simulink model "as_workflow"  (R2021b)
settings: Solver=FixedStepDiscrete  StartTime=0.0  StopTime=inf  FixedStep=0.1  RelTol=1e-3  EnableMultiTasking=on
model workspace (MAT data in the model file):
  Numeric = Simulink.NumericType
  Numeric.DataTypeMode = 'Double'
  Numeric.SignednessBool = 1
  Numeric.WordLength = 64
  Numeric.FixedExponent = 0
  Numeric.SlopeAdjustmentFactor = 1
  Numeric.Bias = 0
  Numeric.DataTypeOverride = 'Inherit'
  Numeric.IsAlias = 1
  Numeric.DataScope = 'Auto'
  Param = Simulink.Parameter
  Param.DataType = 'auto'
  Param.Complexity = 'real'
  Param.Dimensions = [0 0]
  Var = 0
settings Model: DataDictionary=data_state.sldd  Creator=altrof  LastModifiedBy=altrof
settings SolverCC: AlgebraicLoopSolver=TrustRegion  AutoInsertRateTranBlk=on
settings DataIOCC: LimitDataPoints=on
settings OptimizationCC: DefaultParameterBehavior=Inlined  EnhancedBackFolding=on  PassReuseOutputArgsAs=Individual arguments  ZeroExternalMemoryAtStartup=off  ZeroInternalMemoryAtStartup=off  OptimizeBlockOrder=speed  DifferentSizesBufferReuse=on  OptimizationCustomize=off  EfficientTunableParamExpr=on
settings DebuggingCC: ParameterTunabilityLossMsg=error  AllowSymbolicDim=off  SFUnexpectedBacktrackingDiag=warning  SFNoUnconditionalDefaultTransitionDiag=warning  SFExecutionAtInitializationDiag=none  ArithmeticOperatorsInVariantConditions=warning
settings SFSimCC: SimUseLocalCustomCode=off  SimDebugExecutionForCustomCode=on  MATLABDynamicMemAlloc=off  CustomCodeUndefinedFunction=UseInterfaceOnly  CustomCodeGlobalsAsFunctionIO=on  DefaultCustomCodeDeterministicFunctions=All  SimTargetLang=C++
settings RTWCC: Description=Embedded Coder  SystemTargetFile=ert.tlc  GenCodeOnly=on  TemplateMakefile=ert_default_tmf  RTWUseLocalCustomCode=off  TargetLang=C++
settings CodeAppCC: ForceParamTrailComments=on  IgnoreCustomStorageClasses=off  OperatorAnnotations=on  SimulinkDataObjDesc=on  SFDataObjDesc=on  InsertBlockDesc=on  UseSimReservedNames=on
settings ERTTargetCC: TargetLangStandard=C++11 (ISO)  GenerateSampleERTMain=on  CodeInterfacePackaging=C++ class  InlinedParameterPlacement=NonHierarchical  RootIOFormat=Structure reference  ERTCustomFileTemplate=example_file_process.tlc
settings ConfigComp: CovMetricSettings=dw  CovSaveCumulativeToWorkspaceVar=on  CovSaveSingleToWorkspaceVar=on  CovExternalEMLEnable=off  CovSFcnEnable=off

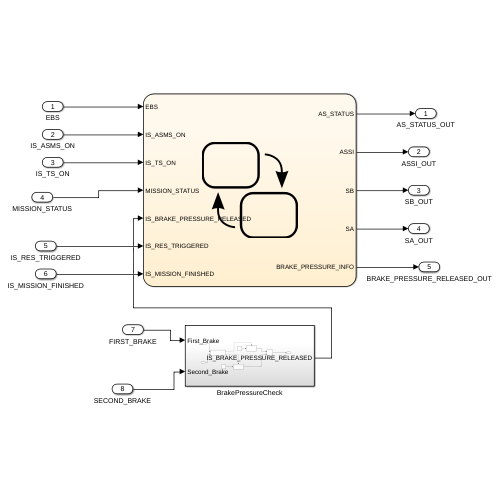
[thumbnail: Simulink's stored preview of the top-level diagram]
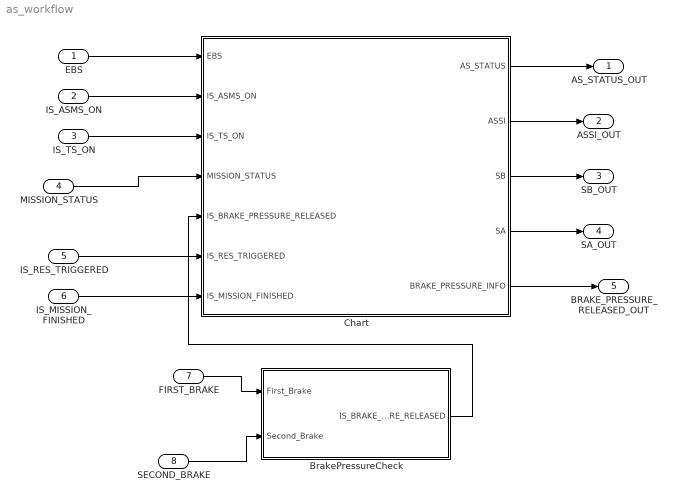
== system as_workflow ==
  EBS : Inport
  IS_ASMS_ON : Inport  Port=2
  IS_TS_ON : Inport  Port=3
  MISSION_STATUS : Inport  Port=4
  IS_RES_TRIGGERED : Inport  Port=5  OutDataTypeStr=boolean
  IS_MISSION_FINISHED : Inport  Port=6  OutDataTypeStr=boolean
  FIRST_BRAKE : Inport  Port=7  OutDataTypeStr=double
  SECOND_BRAKE : Inport  Port=8  OutDataTypeStr=double
  BrakePressureCheck : Subsystem
  Chart : Stateflow chart  TreatAsAtomicUnit=on
  AS_STATUS_OUT : Outport
  ASSI_OUT : Outport  Port=2
  SB_OUT : Outport  Port=3
  SA_OUT : Outport  Port=4
  BRAKE_PRESSURE_RELEASED_OUT : Outport  Port=5
  wires:
  MISSION_STATUS/1 -> Chart/4(MISSION_STATUS)
  EBS/1 -> Chart/1(EBS)
  Chart/1(AS_STATUS) -> AS_STATUS_OUT/1
  Chart/2(ASSI) -> ASSI_OUT/1
  Chart/4(SA) -> SA_OUT/1
  Chart/3(SB) -> SB_OUT/1
  BrakePressureCheck/1(IS_BRAKE_PRESSURE_RELEASED) -> Chart/5(IS_BRAKE_PRESSURE_RELEASED)
  FIRST_BRAKE/1 -> BrakePressureCheck/1(First_Brake)
  SECOND_BRAKE/1 -> BrakePressureCheck/2(Second_Brake)
  Chart/5(BRAKE_PRESSURE_INFO) -> BRAKE_PRESSURE_RELEASED_OUT/1
  IS_RES_TRIGGERED/1 -> Chart/6(IS_RES_TRIGGERED)
  IS_MISSION_FINISHED/1 -> Chart/7(IS_MISSION_FINISHED)
  IS_ASMS_ON/1 -> Chart/2(IS_ASMS_ON)
  IS_TS_ON/1 -> Chart/3(IS_TS_ON)

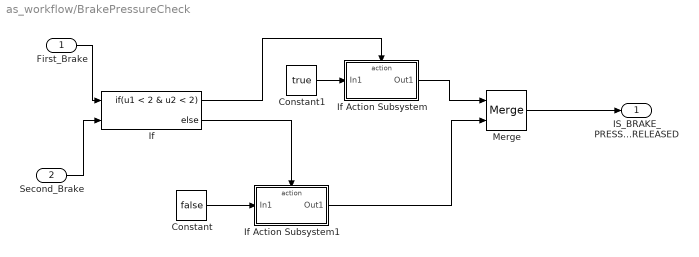
== system as_workflow/BrakePressureCheck ==
  First_Brake : Inport  OutDataTypeStr=double  PortDimensions=1
  Second_Brake : Inport  Port=2  OutDataTypeStr=double  PortDimensions=1
  Constant : Constant  Value=false  OutDataTypeStr=boolean
  Constant1 : Constant  Value=true  OutDataTypeStr=boolean
  If : If  NumInputs=2  IfExpression=u1 < 2 & u2 < 2
  If Action Subsystem : Subsystem  TreatAsAtomicUnit=on
  If Action Subsystem1 : Subsystem  TreatAsAtomicUnit=on
  Merge : Merge
  IS_BRAKE_PRESSURE_RELEASED : Outport
  wires:
  If/1 -> If Action Subsystem/Action
  If/2 -> If Action Subsystem1/Action
  Merge/1 -> IS_BRAKE_PRESSURE_RELEASED/1
  Second_Brake/1 -> If/2
  First_Brake/1 -> If/1
  If Action Subsystem/1(Out1) -> Merge/1
  If Action Subsystem1/1(Out1) -> Merge/2
  Constant/1 -> If Action Subsystem1/1(In1)
  Constant1/1 -> If Action Subsystem/1(In1)

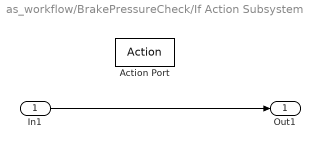
== system as_workflow/BrakePressureCheck/If Action Subsystem ==
  In1 : Inport
  Action Port : ActionPort  ActionPortLabel=if(u1 < 2 & u2 < 2)
  Out1 : Outport
  wires:
  In1/1 -> Out1/1

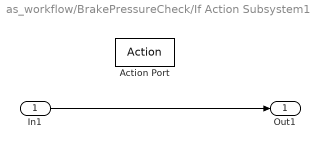
== system as_workflow/BrakePressureCheck/If Action Subsystem1 ==
  In1 : Inport
  Action Port : ActionPort  ActionPortLabel=else
  Out1 : Outport
  wires:
  In1/1 -> Out1/1

== stateflow chart as_workflow/Chart ==
  state AS_READY
    during:
    AS_STATUS = AS_STATE.AS_READY
    SA = SA_STATE.AVAILABLE;
    SB = SB_STATE.ENGAGED;
    ASSI = ASSI_STATE.READY;
  state AS_DRIVING
    during:
    AS_STATUS = AS_STATE.AS_DRIVING
    SA = SA_STATE.AVAILABLE;
    SB = SB_STATE.AVAILABLE;
    ASSI = ASSI_STATE.DRIVING;
  state MANUAL_DRIVING
    during:
    AS_STATUS = AS_STATE.MANUAL
    SA = SA_STATE.UNAVAILABLE;
    SB = SB_STATE.UNAVAILABLE;
    ASSI = ASSI_STATE.OFF;
  state AS_OFF
    during:
    AS_STATUS = AS_STATE.AS_OFF
    SA = SA_STATE.UNAVAILABLE;
    SB = SB_STATE.UNAVAILABLE;
    ASSI = ASSI_STATE.OFF;
    BRAKE_PRESSURE_INFO = IS_BRAKE_PRESSURE_RELEASED
  state AS_EMERGENCY
    during:
    AS_STATUS = AS_STATE.AS_EMERGENCY;
    ASSI = ASSI_STATE.EMERGENCY;
  state AS_FINISHED
    during:
    AS_STATUS = AS_STATE.AS_FINISHED
    SA = SA_STATE.UNAVAILABLE;
    ASSI = ASSI_STATE.FINISHED;
  AS_DRIVING -> AS_FINISHED [order 2] : [IS_MISSION_FINISHED]
  AS_READY -> (junction 63) [order 2] : after(5,sec)
  (junction 63) -> AS_DRIVING
  AS_READY -> AS_EMERGENCY [order 3] : [EBS == EBS_STATE.ACTIVATED]
  AS_OFF -> AS_READY [order 2] : [EBS == EBS_STATE.ARMED && ...
      | MISSION_STATUS == MISSION.AUTONOMOUS && ...
      | IS_TS_ON && IS_ASMS_ON]
  AS_READY -> AS_OFF [order 1] : [~IS_ASMS_ON && ...
      |  IS_BRAKE_PRESSURE_RELEASED]
  AS_DRIVING -> AS_EMERGENCY [order 1] : [EBS == EBS_STATE.ACTIVATED]
  MANUAL_DRIVING -> AS_OFF : [~IS_TS_ON]
  AS_EMERGENCY -> AS_OFF : [~IS_ASMS_ON && ...
      |  IS_BRAKE_PRESSURE_RELEASED]
  AS_FINISHED -> AS_EMERGENCY [order 1] : [IS_RES_TRIGGERED]
  AS_OFF -> MANUAL_DRIVING [order 1] : [MISSION_STATUS == MISSION.MANUAL ...
      | && IS_TS_ON && ~IS_ASMS_ON]
  AS_FINISHED -> AS_OFF [order 2] : [~IS_ASMS_ON && ...
      | IS_BRAKE_PRESSURE_RELEASED]
  (default) -> AS_OFF
  data: EBS input Enum: EBS_STATE; IS_ASMS_ON input boolean; IS_TS_ON input boolean; MISSION_STATUS input Enum: MISSION; AS_STATUS output; ASSI output Enum: ASSI_STATE; SB output Enum: SB_STATE; SA output Enum: SA_STATE; IS_BRAKE_PRESSURE_RELEASED input; BRAKE_PRESSURE_INFO output boolean; IS_RES_TRIGGERED input; IS_MISSION_FINISHED input
